simulink model "prelab1"  (R2020a)
settings: Solver=VariableStepAuto  StartTime=0.0  StopTime=10.0  RelTol=1e-3
values from neighbouring files (symbols this model uses):
  backEmfConstant = 1/s    [transferFunctionsDef.m]
  mechanicalBlock = 1/s    [transferFunctionsDef.m]
  motorConstant = 1/s    [transferFunctionsDef.m]
  pWMAmplifier = 1/s    [transferFunctionsDef.m]
libraries: cstblocks x19, prelab1Library x6
settings Model: Creator=brucecui  LastModifiedBy=brucecui

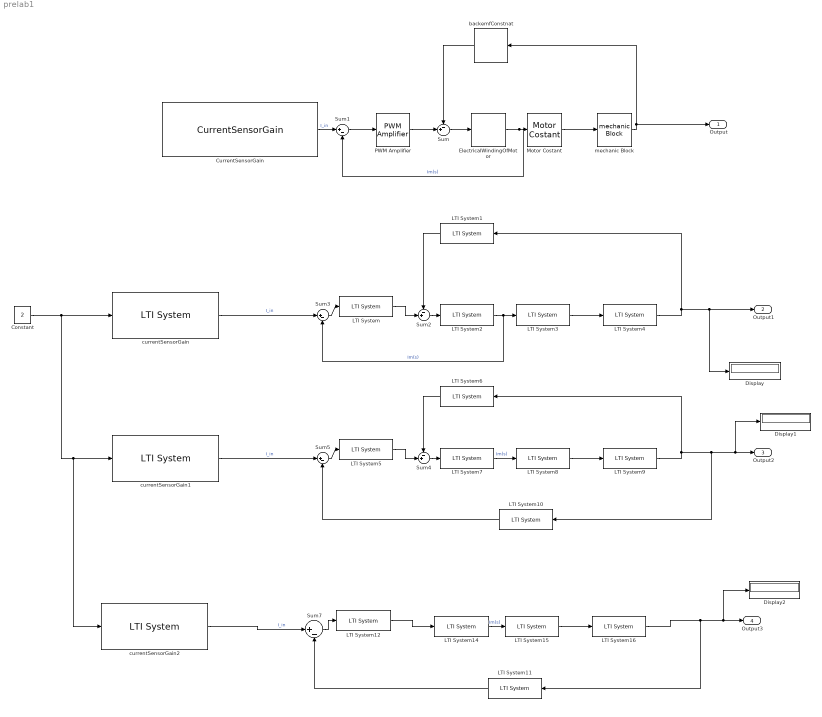
== system prelab1 ==
  Constant : Constant  Value=2
  CurrentSensorGain : prelab1Library/CurrentSensorGain  SystemSampleTime=-1  Latency=0  AutoFrameSizeCalculation=off
  Display : Display
  Display1 : Display
  Display2 : Display
  ElectricalWindingOfMotor : prelab1Library/ElectricalWindingOfMotor  SystemSampleTime=-1  Latency=0  AutoFrameSizeCalculation=off
  LTI System : cstblocks/LTI System  sys=pWMAmplifier  IC=[]
  LTI System1 : cstblocks/LTI System  sys=backEmfConstant  IC=[]
  LTI System10 : cstblocks/LTI System  sys=1/(motorConstant*mechanicalBlock)  IC=[]
  LTI System11 : cstblocks/LTI System  sys=1/(motorConstant*mechanicalBlock) + (backEmfConstant/pWMAmplifier)  IC=[]
  LTI System12 : cstblocks/LTI System  sys=pWMAmplifier  IC=[]
  LTI System14 : cstblocks/LTI System  sys=electricalWindingOfMotor  IC=[]
  LTI System15 : cstblocks/LTI System  sys=motorConstant  IC=[]
  LTI System16 : cstblocks/LTI System  sys=mechanicalBlock  IC=[]
  LTI System2 : cstblocks/LTI System  sys=electricalWindingOfMotor  IC=[]
  LTI System3 : cstblocks/LTI System  sys=motorConstant  IC=[]
  LTI System4 : cstblocks/LTI System  sys=mechanicalBlock  IC=[]
  LTI System5 : cstblocks/LTI System  sys=pWMAmplifier  IC=[]
  LTI System6 : cstblocks/LTI System  sys=backEmfConstant  IC=[]
  LTI System7 : cstblocks/LTI System  sys=electricalWindingOfMotor  IC=[]
  LTI System8 : cstblocks/LTI System  sys=motorConstant  IC=[]
  LTI System9 : cstblocks/LTI System  sys=mechanicalBlock  IC=[]
  Motor Costant : prelab1Library/Motor Costant  SystemSampleTime=-1  Latency=0  AutoFrameSizeCalculation=off
  PWM Amplifier : prelab1Library/PWM Amplifier  SystemSampleTime=-1  Latency=0  AutoFrameSizeCalculation=off
  Sum : Sum  Inputs=-+|
  Sum{1,3,5,7} (4 alike) : Sum  Inputs=|+-
  Sum2 : Sum  Inputs=-+|
  Sum4 : Sum  Inputs=-+|
  backemfConstnat : prelab1Library/backemfConstnat  SystemSampleTime=-1  Latency=0  AutoFrameSizeCalculation=off
  currentSensorGain : cstblocks/LTI System  sys=currentSensorGain  IC=[]
  currentSensorGain1 : cstblocks/LTI System  sys=currentSensorGain  IC=[]
  currentSensorGain2 : cstblocks/LTI System  sys=currentSensorGain  IC=[]
  mechanic Block : prelab1Library/mechanic Block  SystemSampleTime=-1  Latency=0  AutoFrameSizeCalculation=off
  Output : Outport
  Output1 : Outport  Port=2
  Output2 : Outport  Port=3
  Output3 : Outport  Port=4
  wires:
  PWM Amplifier/1 -> Sum/2
  ElectricalWindingOfMotor/1 -> Sum1/2, Motor Costant/1  "Im(s)"
  Motor Costant/1 -> mechanic Block/1
  backemfConstnat/1 -> Sum/1
  CurrentSensorGain/1 -> Sum1/1  "I_in"
  mechanic Block/1 -> Output/1, backemfConstnat/1
  Sum/1 -> ElectricalWindingOfMotor/1
  Sum1/1 -> PWM Amplifier/1
  LTI System4/1 -> LTI System1/1, Display/1, Output1/1
  LTI System2/1 -> Sum3/2, LTI System3/1  "Im(s)"
  LTI System/1 -> Sum2/2
  LTI System3/1 -> LTI System4/1
  Sum2/1 -> LTI System2/1
  LTI System1/1 -> Sum2/1
  currentSensorGain/1 -> Sum3/1  "I_in"
  Sum3/1 -> LTI System/1
  currentSensorGain1/1 -> Sum5/1  "I_in"
  LTI System8/1 -> LTI System9/1
  Sum5/1 -> LTI System5/1
  LTI System6/1 -> Sum4/1
  LTI System5/1 -> Sum4/2
  LTI System7/1 -> LTI System8/1  "Im(s)"
  Sum4/1 -> LTI System7/1
  LTI System9/1 -> LTI System6/1, LTI System10/1, Display1/1, Output2/1
  LTI System10/1 -> Sum5/2
  Constant/1 -> currentSensorGain2/1, currentSensorGain1/1, currentSensorGain/1
  LTI System11/1 -> Sum7/2
  LTI System14/1 -> LTI System15/1  "Im(s)"
  currentSensorGain2/1 -> Sum7/1  "I_in"
  LTI System15/1 -> LTI System16/1
  Sum7/1 -> LTI System12/1
  LTI System16/1 -> LTI System11/1, Display2/1, Output3/1
  LTI System12/1 -> LTI System14/1
